simulink model "ES105A_StHlthSigNormn"  (R2013b)
settings: Solver=FixedStepDiscrete  SolverMode=SingleTasking  StartTime=0.0  StopTime=1  FixedStep=0.002  RelTol=1e-3
undefined symbols (not defined in the file): ARCHGLBPRM_FLOATZEROTHD_ULS_F32, CurrMeasCorrlnMaxErrCurr, CURRMOTSUMDIVBYZEROPROTNVAL_AMPR_F32, DIGTQDIVBYZEROPROTNVAL_HWNWTMTR_F32, DutyCycThermProtnDutyCycFildThd, EcuTMeasRngDiagcMax, EcuTMeasRngDiagcMin, EotLrngAuthyStrtLrn, FRICESTIMNDIVBYZEROPROTNVAL_HWNWTMTR_F32, HLTH0PERC_CNT_U08, HLTH100PERC_CNT_F32, HLTH100PERC_CNT_U08, HLTH50PERC_CNT_U08, HwTqCorrlnChATraSumSetFltThd, HwTqCorrlnChBTraSumSetFltThd, HWTQIDPTSIG_CNT_U08, MOTAG2MEAS_VALMAXERR_VOLTSQD_F32, MOTAG2MEAS_VALMINERR_VOLTSQD_F32, MOTAGCORRLN_MOTAGCORRLNERRTHD_MOTREVELEC_U0P16, MotDrvDiagcErrThd, MOTPOS2DIVBYZEROPROTNVAL2_VOLTSQD_F32, MOTPOS2DIVBYZEROPROTNVAL_VOLTSQD_F32, MOTPOSNERRDIVBYZEROPROTNVAL_MOTREV_U16, MOTPOSNERRZEROTHD_MOTREV_U0P16, NtcNr1, NtcSts1, PHAVLTGDIVBYZEROPROTNVAL_NANOSEC_F32, SigQlfr1, STHLTHSCAGFAC_CNT_F32, StHlthSigNormnAbsltMotPosDifStHlthDiagThd, StHlthSigNormnCurrMotSumStHlthDiagThd, StHlthSigNormnDigTqStHlthDiagThd, StHlthSigNormnDutyCycFltLimThd, StHlthSigNormnHiCtrlrT, StHlthSigNormnIdptSigStHlthSca, StHlthSigNormnLoCtrlrT, StHlthSigNormnMaxFricThd, StHlthSigNormnMinRackTrvlLim, StHlthSigNormnMotPosStHlthDiagThd, StHlthSigNormnMotVelCal, StHlthSigNormnPhaInfoStHlthDiagThd, StHlthSigNormnStHlthCorrlnErr, StHlthSigNormnStHlthCurrMotSum, StHlthSigNormnStHlthPhaInfo, StHlthSigNormnValMaxStHlthErr, StHlthSigNormnValMinStHlthErr, StHlthSigNormnWhlImbRejctnThd, SysGlbPrmMotPoleCnt, TSTHLTH0PERC_CNT_U08, u2, u3, u4, VLTGSTHLTH0PERC_CNT_U08
libraries: NxtrLim x39, simulink x33, NxtrAbslt x4
(part 3 of 10)

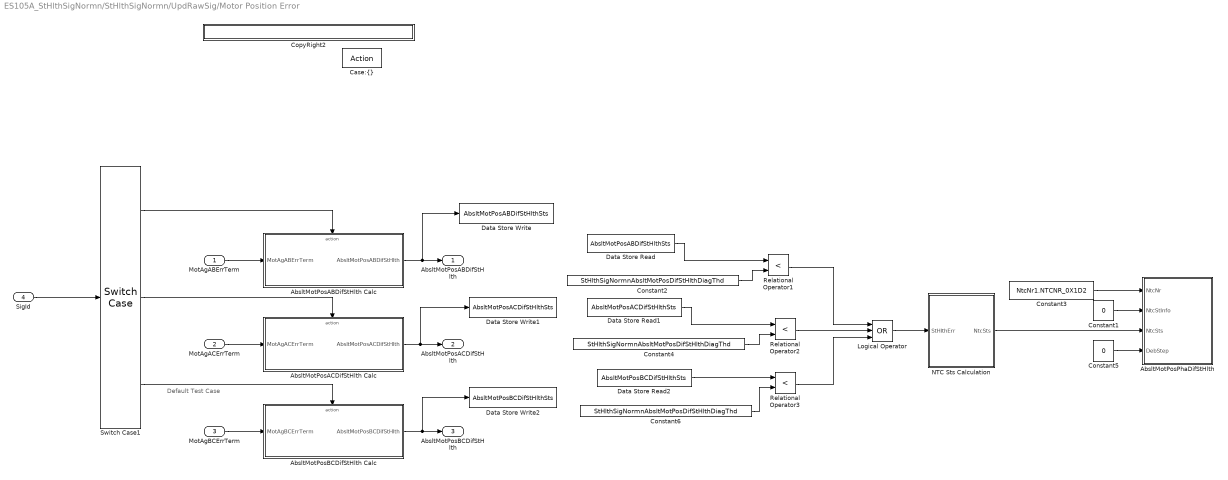
== system ES105A_StHlthSigNormn/StHlthSigNormn/UpdRawSig/Motor Position Error  ==
  note: Default Test Case
  MotAgABErrTerm : Inport
  MotAgACErrTerm : Inport  Port=2
  MotAgBCErrTerm : Inport  Port=3
  SigId : Inport  Port=4
  "Case:{}" : ActionPort  ActionType=case
  AbsltMotPosABDifStHlth Calc : Subsystem  TreatAsAtomicUnit=on
  AbsltMotPosACDifStHlth Calc : Subsystem  TreatAsAtomicUnit=on
  AbsltMotPosBCDifStHlth Calc : Subsystem  TreatAsAtomicUnit=on
  AbsltMotPosPhaDifStHlth : Subsystem  mask(SetNTC){}
      mask help: SetNTC library block
  Constant1 : Constant  Value=0  OutDataTypeStr=uint8
      settings: AttributesFormatString=%<OutDataTypeStr>
  Constant2 : Constant  Value=StHlthSigNormnAbsltMotPosDifStHlthDiagThd
  Constant3 : Constant  Value=NtcNr1.NTCNR_0X1D2  OutDataTypeStr=Enum: NtcNr1
  Constant4 : Constant  Value=StHlthSigNormnAbsltMotPosDifStHlthDiagThd
  Constant5 : Constant  Value=0  OutDataTypeStr=uint16
      settings: AttributesFormatString=%<OutDataTypeStr>
  Constant6 : Constant  Value=StHlthSigNormnAbsltMotPosDifStHlthDiagThd
  CopyRight2 : Subsystem  Description=|  mask(Copyright Information){none=on}
      | Copyright info block.                                               
      |                                                                     
      | Place copyright information at the top of every subsystem in design.
      mask prompts: none "No parameters"
      mask help: Place copyright information at the top of every subsystem in design.
      mask Display:
      | NxtrConf = 'Nexteer Confidential';
      | 
      | sys = bdroot; %handle for the current model ("system")
      | first = get_param(sys,'Created');
      | first = first(end-3:end);  %year is last four digits
      | 
      | last = get_param(sys,'LastModifiedDate');
      | if isempty(last)
      |     last = datestr(now,'yyyy');
      | else
      |     last = last(end-3:end);
      | end
      | 
      | if strcmp(first,last)
      |     fprintf('%s -- Copyright %s Nexteer',NxtrConf,first)
      | else
      |     fprintf('%s -- %s%s- %s Nexteer',NxtrConf,char(169),first,last)
      | end
  Data Store Read : DataStoreRead  DataStoreName=AbsltMotPosABDifStHlthSts
  Data Store Read1 : DataStoreRead  DataStoreName=AbsltMotPosACDifStHlthSts
  Data Store Read2 : DataStoreRead  DataStoreName=AbsltMotPosBCDifStHlthSts
  Data Store Write : DataStoreWrite  DataStoreName=AbsltMotPosABDifStHlthSts
  Data Store Write1 : DataStoreWrite  DataStoreName=AbsltMotPosACDifStHlthSts
  Data Store Write2 : DataStoreWrite  DataStoreName=AbsltMotPosBCDifStHlthSts
  Logical Operator : Logic  Operator=OR  Inputs=3  AllPortsSameDT=off  OutDataTypeStr=boolean
  NTC Sts Calculation : Subsystem
  Relational Operator1 : RelationalOperator  Operator=<  OutDataTypeStr=boolean
  Relational Operator2 : RelationalOperator  Operator=<  OutDataTypeStr=boolean
  Relational Operator3 : RelationalOperator  Operator=<  OutDataTypeStr=boolean
  Switch Case1 : SwitchCase  CaseConditions={StHlthMonSig3.STHLTHMONSIG_MOTPOSABDIFF, StHlthMonSig3.STHLTHMONSIG_MOTPOSACDIFF}
  AbsltMotPosABDifStHlth : Outport
  AbsltMotPosACDifStHlth : Outport  Port=2
  AbsltMotPosBCDifStHlth : Outport  Port=3
  wires:
  Constant3/1 -> AbsltMotPosPhaDifStHlth/1(NtcNr)
  Constant1/1 -> AbsltMotPosPhaDifStHlth/2(NtcStInfo)
  Constant5/1 -> AbsltMotPosPhaDifStHlth/4(DebStep)
  NTC Sts Calculation/1(NtcSts) -> AbsltMotPosPhaDifStHlth/3(NtcSts)
  AbsltMotPosACDifStHlth Calc/1(AbsltMotPosACDifStHlth) -> Data Store Write1/1, AbsltMotPosACDifStHlth/1
  Switch Case1/1 -> AbsltMotPosABDifStHlth Calc/Action
  MotAgABErrTerm/1 -> AbsltMotPosABDifStHlth Calc/1(MotAgABErrTerm)
  Switch Case1/2 -> AbsltMotPosACDifStHlth Calc/Action
  MotAgACErrTerm/1 -> AbsltMotPosACDifStHlth Calc/1(MotAgACErrTerm)
  Switch Case1/3 -> AbsltMotPosBCDifStHlth Calc/Action
  MotAgBCErrTerm/1 -> AbsltMotPosBCDifStHlth Calc/1(MotAgBCErrTerm)
  SigId/1 -> Switch Case1/1
  AbsltMotPosABDifStHlth Calc/1(AbsltMotPosABDifStHlth) -> Data Store Write/1, AbsltMotPosABDifStHlth/1
  AbsltMotPosBCDifStHlth Calc/1(AbsltMotPosBCDifStHlth) -> Data Store Write2/1, AbsltMotPosBCDifStHlth/1
  Constant2/1 -> Relational Operator1/2
  Data Store Read/1 -> Relational Operator1/1
  Constant4/1 -> Relational Operator2/2
  Data Store Read1/1 -> Relational Operator2/1
  Constant6/1 -> Relational Operator3/2
  Data Store Read2/1 -> Relational Operator3/1
  Relational Operator1/1 -> Logical Operator/1
  Relational Operator2/1 -> Logical Operator/2
  Relational Operator3/1 -> Logical Operator/3
  Logical Operator/1 -> NTC Sts Calculation/1(StHlthErr)

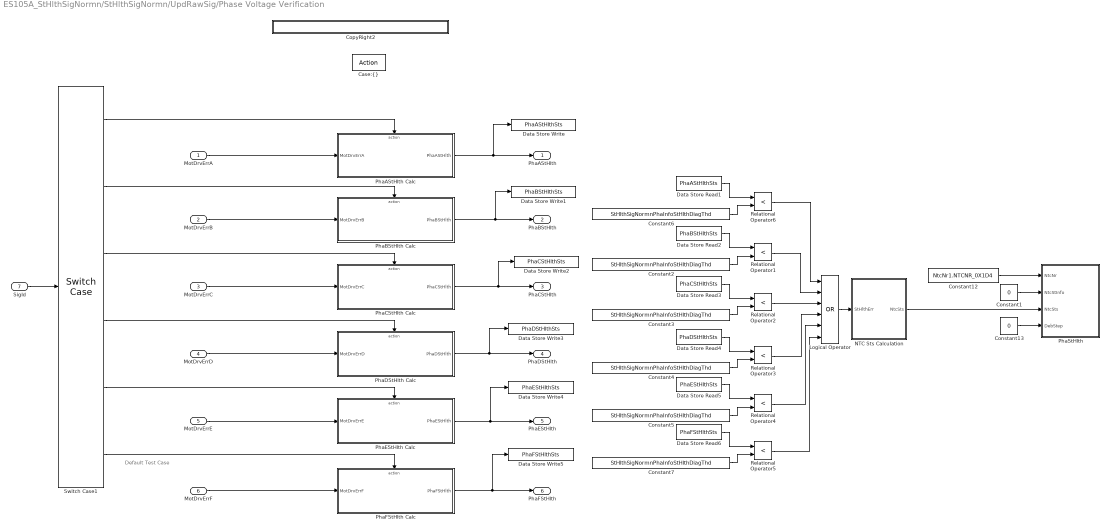
== system ES105A_StHlthSigNormn/StHlthSigNormn/UpdRawSig/Phase Voltage Verification ==
  note: Default Test Case
  MotDrvErrA : Inport
  MotDrvErrB : Inport  Port=2
  MotDrvErrC : Inport  Port=3
  MotDrvErrD : Inport  Port=4
  MotDrvErrE : Inport  Port=5
  MotDrvErrF : Inport  Port=6
  SigId : Inport  Port=7
  "Case:{}" : ActionPort  ActionType=case
  Constant1 : Constant  Value=0  OutDataTypeStr=uint8
      settings: AttributesFormatString=%<OutDataTypeStr>
  Constant12 : Constant  Value=NtcNr1.NTCNR_0X1D4  OutDataTypeStr=Enum: NtcNr1
  Constant13 : Constant  Value=0  OutDataTypeStr=uint16
      settings: AttributesFormatString=%<OutDataTypeStr>
  Constant{2..7} (6 alike) : Constant  Value=StHlthSigNormnPhaInfoStHlthDiagThd
  CopyRight2 : Subsystem  Description=|  mask(Copyright Information){none=on}
      | Copyright info block.                                               
      |                                                                     
      | Place copyright information at the top of every subsystem in design.
      mask prompts: none "No parameters"
      mask help: Place copyright information at the top of every subsystem in design.
      mask Display:
      | NxtrConf = 'Nexteer Confidential';
      | 
      | sys = bdroot; %handle for the current model ("system")
      | first = get_param(sys,'Created');
      | first = first(end-3:end);  %year is last four digits
      | 
      | last = get_param(sys,'LastModifiedDate');
      | if isempty(last)
      |     last = datestr(now,'yyyy');
      | else
      |     last = last(end-3:end);
      | end
      | 
      | if strcmp(first,last)
      |     fprintf('%s -- Copyright %s Nexteer',NxtrConf,first)
      | else
      |     fprintf('%s -- %s%s- %s Nexteer',NxtrConf,char(169),first,last)
      | end
  Data Store Read1 : DataStoreRead  DataStoreName=PhaAStHlthSts
  Data Store Read2 : DataStoreRead  DataStoreName=PhaBStHlthSts
  Data Store Read3 : DataStoreRead  DataStoreName=PhaCStHlthSts
  Data Store Read4 : DataStoreRead  DataStoreName=PhaDStHlthSts
  Data Store Read5 : DataStoreRead  DataStoreName=PhaEStHlthSts
  Data Store Read6 : DataStoreRead  DataStoreName=PhaFStHlthSts
  Data Store Write : DataStoreWrite  DataStoreName=PhaAStHlthSts
  Data Store Write1 : DataStoreWrite  DataStoreName=PhaBStHlthSts
  Data Store Write2 : DataStoreWrite  DataStoreName=PhaCStHlthSts
  Data Store Write3 : DataStoreWrite  DataStoreName=PhaDStHlthSts
  Data Store Write4 : DataStoreWrite  DataStoreName=PhaEStHlthSts
  Data Store Write5 : DataStoreWrite  DataStoreName=PhaFStHlthSts
  Logical Operator : Logic  Operator=OR  Inputs=6  AllPortsSameDT=off  OutDataTypeStr=boolean
  NTC Sts Calculation : Subsystem
  PhaAStHlth Calc : Subsystem  TreatAsAtomicUnit=on
  PhaBStHlth Calc : Subsystem  TreatAsAtomicUnit=on
  PhaCStHlth Calc : Subsystem  TreatAsAtomicUnit=on
  PhaDStHlth Calc : Subsystem  TreatAsAtomicUnit=on
  PhaEStHlth Calc : Subsystem  TreatAsAtomicUnit=on
  PhaFStHlth Calc : Subsystem  TreatAsAtomicUnit=on
  PhaStHlth : Subsystem  mask(SetNTC){}
      mask help: SetNTC library block
  Relational Operator{1..6} (6 alike) : RelationalOperator  Operator=<  OutDataTypeStr=boolean
  Switch Case1 : SwitchCase  CaseConditions={StHlthMonSig3.STHLTHMONSIG_MOTPOSPHASEA,StHlthMonSig3.STHLTHMONSIG_MOTPOSPHASEB,StHlthMonSig3.STHLTHMONSIG_MOTPOSPHASEC,StHlthMonSig3.STHLTHMONSIG_MOTPOSPHASED,StHlthMonSig3.STHLTHMONSIG_MOTPOSPHASEE}
  PhaAStHlth : Outport
  PhaBStHlth : Outport  Port=2
  PhaCStHlth : Outport  Port=3
  PhaDStHlth : Outport  Port=4
  PhaEStHlth : Outport  Port=5
  PhaFStHlth : Outport  Port=6
  wires:
  Constant12/1 -> PhaStHlth/1(NtcNr)
  Constant1/1 -> PhaStHlth/2(NtcStInfo)
  Constant13/1 -> PhaStHlth/4(DebStep)
  NTC Sts Calculation/1(NtcSts) -> PhaStHlth/3(NtcSts)
  MotDrvErrA/1 -> PhaAStHlth Calc/1(MotDrvErrA)
  MotDrvErrB/1 -> PhaBStHlth Calc/1(MotDrvErrB)
  MotDrvErrC/1 -> PhaCStHlth Calc/1(MotDrvErrC)
  MotDrvErrD/1 -> PhaDStHlth Calc/1(MotDrvErrD)
  MotDrvErrE/1 -> PhaEStHlth Calc/1(MotDrvErrE)
  MotDrvErrF/1 -> PhaFStHlth Calc/1(MotDrvErrF)
  Switch Case1/1 -> PhaAStHlth Calc/Action
  Switch Case1/2 -> PhaBStHlth Calc/Action
  Switch Case1/3 -> PhaCStHlth Calc/Action
  Switch Case1/4 -> PhaDStHlth Calc/Action
  Switch Case1/5 -> PhaEStHlth Calc/Action
  Switch Case1/6 -> PhaFStHlth Calc/Action
  SigId/1 -> Switch Case1/1
  PhaEStHlth Calc/1(PhaEStHlth) -> Data Store Write4/1, PhaEStHlth/1
  PhaAStHlth Calc/1(PhaAStHlth) -> Data Store Write/1, PhaAStHlth/1
  PhaBStHlth Calc/1(PhaBStHlth) -> Data Store Write1/1, PhaBStHlth/1
  PhaCStHlth Calc/1(PhaCStHlth) -> Data Store Write2/1, PhaCStHlth/1
  PhaDStHlth Calc/1(PhaDStHlth) -> Data Store Write3/1, PhaDStHlth/1
  PhaFStHlth Calc/1(PhaFStHlth) -> Data Store Write5/1, PhaFStHlth/1
  Constant6/1 -> Relational Operator6/2
  Data Store Read1/1 -> Relational Operator6/1
  Constant2/1 -> Relational Operator1/2
  Data Store Read2/1 -> Relational Operator1/1
  Constant3/1 -> Relational Operator2/2
  Data Store Read3/1 -> Relational Operator2/1
  Constant4/1 -> Relational Operator3/2
  Data Store Read4/1 -> Relational Operator3/1
  Constant5/1 -> Relational Operator4/2
  Data Store Read5/1 -> Relational Operator4/1
  Constant7/1 -> Relational Operator5/2
  Data Store Read6/1 -> Relational Operator5/1
  Relational Operator1/1 -> Logical Operator/2
  Relational Operator6/1 -> Logical Operator/1
  Relational Operator2/1 -> Logical Operator/3
  Relational Operator3/1 -> Logical Operator/4
  Relational Operator4/1 -> Logical Operator/5
  Relational Operator5/1 -> Logical Operator/6
  Logical Operator/1 -> NTC Sts Calculation/1(StHlthErr)

== system ES105A_StHlthSigNormn/StHlthSigNormn/UpdRawSig/Single Bit Correction  ==
  note: Datatype conversion is added to avoid simulation error as
      | Uint8 is expected at the input of saturation block
  LclRamEccSngBitCntrOutp : Inport
  "Case:{}" : ActionPort  ActionType=case
  Constant : Constant  Value=STHLTHSCAGFAC_CNT_F32  OutDataTypeStr=single
  CopyRight2 : Subsystem  Description=|  mask(Copyright Information){none=on}
      | Copyright info block.                                               
      |                                                                     
      | Place copyright information at the top of every subsystem in design.
      mask prompts: none "No parameters"
      mask help: Place copyright information at the top of every subsystem in design.
      mask Display:
      | NxtrConf = 'Nexteer Confidential';
      | 
      | sys = bdroot; %handle for the current model ("system")
      | first = get_param(sys,'Created');
      | first = first(end-3:end);  %year is last four digits
      | 
      | last = get_param(sys,'LastModifiedDate');
      | if isempty(last)
      |     last = datestr(now,'yyyy');
      | else
      |     last = last(end-3:end);
      | end
      | 
      | if strcmp(first,last)
      |     fprintf('%s -- Copyright %s Nexteer',NxtrConf,first)
      | else
      |     fprintf('%s -- %s%s- %s Nexteer',NxtrConf,char(169),first,last)
      | end
  Data Type Conversion : DataTypeConversion  OutDataTypeStr=uint8
  LimStat_u2 : NxtrLim/LimStat_u08  LoLim=RamEccSngBitCorrnStHlth.EngMin  HiLim=RamEccSngBitCorrnStHlth.EngMax
      settings: AttributesFormatString=|
      | Low Limit: %<LoLim>
      | High Limit:%<HiLim>
  Subtract : Sum  Inputs=+-
  RamEccSngBitCorrnStHlth : Outport
  wires:
  Constant/1 -> Data Type Conversion/1
  LclRamEccSngBitCntrOutp/1 -> Subtract/2
  Subtract/1 -> LimStat_u2/1
  LimStat_u2/1 -> RamEccSngBitCorrnStHlth/1
  Data Type Conversion/1 -> Subtract/1

== system ES105A_StHlthSigNormn/StHlthSigNormn/UpdRawSig/Wheel Imbalance Rejection ==
  WhlImbRejctnCmd : Inport
  "Case:{}" : ActionPort  ActionType=case
  Abs : Abs
  Constant : Constant  Value=StHlthSigNormnWhlImbRejctnThd
  CopyRight2 : Subsystem  Description=|  mask(Copyright Information){none=on}
      | Copyright info block.                                               
      |                                                                     
      | Place copyright information at the top of every subsystem in design.
      mask prompts: none "No parameters"
      mask help: Place copyright information at the top of every subsystem in design.
      mask Display:
      | NxtrConf = 'Nexteer Confidential';
      | 
      | sys = bdroot; %handle for the current model ("system")
      | first = get_param(sys,'Created');
      | first = first(end-3:end);  %year is last four digits
      | 
      | last = get_param(sys,'LastModifiedDate');
      | if isempty(last)
      |     last = datestr(now,'yyyy');
      | else
      |     last = last(end-3:end);
      | end
      | 
      | if strcmp(first,last)
      |     fprintf('%s -- Copyright %s Nexteer',NxtrConf,first)
      | else
      |     fprintf('%s -- %s%s- %s Nexteer',NxtrConf,char(169),first,last)
      | end
  If : If  IfExpression=u1
  If Action Subsystem : Subsystem  TreatAsAtomicUnit=on
  If Action Subsystem2 : Subsystem  TreatAsAtomicUnit=on
  LimStat_u2 : NxtrLim/LimStat_u08  LoLim=WHLIMBMAXCMPSTHLTHLOLI_CNT_U08  HiLim=WHLIMBMAXCMPSTHLTHHILI_CNT_U08
      settings: AttributesFormatString=|
      | Low Limit: %<LoLim>
      | High Limit:%<HiLim>
  Merge : Merge
  Relational Operator : RelationalOperator  OutDataTypeStr=boolean
  WhlImbMaxCmpStHlth : Outport
  wires:
  Constant/1 -> Relational Operator/2
  Relational Operator/1 -> If/1
  If/1 -> If Action Subsystem/Action
  WhlImbRejctnCmd/1 -> Abs/1
  If/2 -> If Action Subsystem2/Action
  If Action Subsystem/1(WhlImbMaxCmpStHlth) -> Merge/1
  If Action Subsystem2/1(WhlImbMaxCmpStHlth) -> Merge/2
  Merge/1 -> LimStat_u2/1
  LimStat_u2/1 -> WhlImbMaxCmpStHlth/1
  Abs/1 -> Relational Operator/1

== system ES105A_StHlthSigNormn/StHlthSigNormn/StHlthSigNormnInit1/GetFricLrngData/CopyRight2 ==

== system ES105A_StHlthSigNormn/StHlthSigNormn/StHlthSigNormnInit1/Motror Angle Threshold Calc/CopyRight2 ==

== system ES105A_StHlthSigNormn/StHlthSigNormn/UpdRawSig/ EOT Impact Counter/CopyRight2 ==

== system ES105A_StHlthSigNormn/StHlthSigNormn/UpdRawSig/ EOT Impact Counter/If Action Subsystem ==
  HwAg : Inport
  RackLimrEotSig0Avl : Inport  Port=2
  MotVelCrf : Inport  Port=3
  HwAgEotCcw : Inport  Port=4
  RackLimrEotSig1Avl : Inport  Port=5
  HwAgEotCw : Inport  Port=6
  Action Port : ActionPort  ActionType=then
  Constant : Constant  Value=ARCHGLBPRM_FLOATZEROTHD_ULS_F32
  CopyRight2 : Subsystem  Description=|  mask(Copyright Information){none=on}
      | Copyright info block.                                               
      |                                                                     
      | Place copyright information at the top of every subsystem in design.
      mask prompts: none "No parameters"
      mask help: Place copyright information at the top of every subsystem in design.
      mask Display:
      | NxtrConf = 'Nexteer Confidential';
      | 
      | sys = bdroot; %handle for the current model ("system")
      | first = get_param(sys,'Created');
      | first = first(end-3:end);  %year is last four digits
      | 
      | last = get_param(sys,'LastModifiedDate');
      | if isempty(last)
      |     last = datestr(now,'yyyy');
      | else
      |     last = last(end-3:end);
      | end
      | 
      | if strcmp(first,last)
      |     fprintf('%s -- Copyright %s Nexteer',NxtrConf,first)
      | else
      |     fprintf('%s -- %s%s- %s Nexteer',NxtrConf,char(169),first,last)
      | end
  If : If  IfExpression=u1
  If Action Subsystem : Subsystem  TreatAsAtomicUnit=on
  If Action Subsystem1 : Subsystem  TreatAsAtomicUnit=on
  Relational Operator : RelationalOperator  OutDataTypeStr=boolean
  wires:
  HwAg/1 -> Relational Operator/1, [HwAg]
  Constant/1 -> Relational Operator/2
  Relational Operator/1 -> If/1
  If/1 -> If Action Subsystem/Action
  RackLimrEotSig1Avl/1 -> If Action Subsystem/1(RackLimrEotSig1Avl)
  HwAgEotCw/1 -> If Action Subsystem/4(HwAgEotCw)
  If/2 -> If Action Subsystem1/Action
  MotVelCrf/1 -> [MotVelCrf], If Action Subsystem1/3(MotVelCrf)
  RackLimrEotSig0Avl/1 -> If Action Subsystem1/1(RackLimrEotSig0Avl)
  HwAgEotCcw/1 -> If Action Subsystem1/4(HwAgEotCcw)
  [MotVelCrf] -> If Action Subsystem/3("MotVelCrf ")
  [HwAg] -> If Action Subsystem/2(HwAg)
  [HwAg] -> If Action Subsystem1/2(HwAg)

== system ES105A_StHlthSigNormn/StHlthSigNormn/UpdRawSig/ EOT Impact Counter/If Action Subsystem1 ==
  Action Port : ActionPort  ActionType=else
  Constant : Constant  Value=0  OutDataTypeStr=boolean
      settings: AttributesFormatString=%<OutDataTypeStr>
  CopyRight2 : Subsystem  Description=|  mask(Copyright Information){none=on}
      | Copyright info block.                                               
      |                                                                     
      | Place copyright information at the top of every subsystem in design.
      mask prompts: none "No parameters"
      mask help: Place copyright information at the top of every subsystem in design.
      mask Display:
      | NxtrConf = 'Nexteer Confidential';
      | 
      | sys = bdroot; %handle for the current model ("system")
      | first = get_param(sys,'Created');
      | first = first(end-3:end);  %year is last four digits
      | 
      | last = get_param(sys,'LastModifiedDate');
      | if isempty(last)
      |     last = datestr(now,'yyyy');
      | else
      |     last = last(end-3:end);
      | end
      | 
      | if strcmp(first,last)
      |     fprintf('%s -- Copyright %s Nexteer',NxtrConf,first)
      | else
      |     fprintf('%s -- %s%s- %s Nexteer',NxtrConf,char(169),first,last)
      | end
  Data Store Write : DataStoreWrite  DataStoreName=EntrEot
  wires:
  Constant/1 -> Data Store Write/1

== system ES105A_StHlthSigNormn/StHlthSigNormn/UpdRawSig/ Health Of Assist Due To Voltage/CopyRight2 ==

== system ES105A_StHlthSigNormn/StHlthSigNormn/UpdRawSig/ Health Of Assist Due To Voltage/Do nothing ==
  Action Port : ActionPort  ActionType=else
  CopyRight2 : Subsystem  Description=|  mask(Copyright Information){none=on}
      | Copyright info block.                                               
      |                                                                     
      | Place copyright information at the top of every subsystem in design.
      mask prompts: none "No parameters"
      mask help: Place copyright information at the top of every subsystem in design.
      mask Display:
      | NxtrConf = 'Nexteer Confidential';
      | 
      | sys = bdroot; %handle for the current model ("system")
      | first = get_param(sys,'Created');
      | first = first(end-3:end);  %year is last four digits
      | 
      | last = get_param(sys,'LastModifiedDate');
      | if isempty(last)
      |     last = datestr(now,'yyyy');
      | else
      |     last = last(end-3:end);
      | end
      | 
      | if strcmp(first,last)
      |     fprintf('%s -- Copyright %s Nexteer',NxtrConf,first)
      | else
      |     fprintf('%s -- %s%s- %s Nexteer',NxtrConf,char(169),first,last)
      | end

== system ES105A_StHlthSigNormn/StHlthSigNormn/UpdRawSig/ Health Of Assist Due To Voltage/LowVoltage ==
  Action Port : ActionPort  ActionType=elseif
  Bitwise Operator : simulink/Logic and Bit Operations/Bitwise Operator  logicop=OR  UseBitMask=off  NumInputPorts=2  BitMask=bin2dec('11011001')  BitMaskRealWorld=Stored Integer
  Constant1 : Constant  Value=HLTH50PERC_CNT_U08  OutDataTypeStr=uint8
  Constant2 : Constant  OutDataTypeStr=uint8
      settings: AttributesFormatString=%<OutDataTypeStr>
  Constant3 : Constant  OutDataTypeStr=uint8
      settings: AttributesFormatString=%<OutDataTypeStr>
  CopyRight2 : Subsystem  Description=|  mask(Copyright Information){none=on}
      | Copyright info block.                                               
      |                                                                     
      | Place copyright information at the top of every subsystem in design.
      mask prompts: none "No parameters"
      mask help: Place copyright information at the top of every subsystem in design.
      mask Display:
      | NxtrConf = 'Nexteer Confidential';
      | 
      | sys = bdroot; %handle for the current model ("system")
      | first = get_param(sys,'Created');
      | first = first(end-3:end);  %year is last four digits
      | 
      | last = get_param(sys,'LastModifiedDate');
      | if isempty(last)
      |     last = datestr(now,'yyyy');
      | else
      |     last = last(end-3:end);
      | end
      | 
      | if strcmp(first,last)
      |     fprintf('%s -- Copyright %s Nexteer',NxtrConf,first)
      | else
      |     fprintf('%s -- %s%s- %s Nexteer',NxtrConf,char(169),first,last)
      | end
  Data Store Read : DataStoreRead  DataStoreName=VltgRngIgnCyc
  Data Store Write : DataStoreWrite  DataStoreName=VltgRngIgnCyc
  Shift Arithmetic : ArithShift  BitShiftNumber=LOVLTGSTHLTH50PERC_CNT_U08  BitShiftDirection=Left
  Shift Arithmetic1 : ArithShift  BitShiftNumber=LOVLTGSTHLTH50PERC_CNT_U08  BitShiftDirection=Left
  OutpAssiStHlth : Outport
  " PrsntVltgRng" : Outport  Port=2
  wires:
  Constant1/1 -> OutpAssiStHlth/1
  Constant2/1 -> Shift Arithmetic/1
  Shift Arithmetic/1 -> Bitwise Operator/2
  Data Store Read/1 -> Bitwise Operator/1
  Bitwise Operator/1 -> Data Store Write/1
  Constant3/1 -> Shift Arithmetic1/1
  Shift Arithmetic1/1 -> " PrsntVltgRng"/1

== system ES105A_StHlthSigNormn/StHlthSigNormn/UpdRawSig/ Health Of Assist Due To Voltage/NtcLoVltgActvSts ==
  NtcNr : Inport
  CopyRight2 : Subsystem  Description=|  mask(Copyright Information){none=on}
      | Copyright info block.                                               
      |                                                                     
      | Place copyright information at the top of every subsystem in design.
      mask prompts: none "No parameters"
      mask help: Place copyright information at the top of every subsystem in design.
      mask Display:
      | NxtrConf = 'Nexteer Confidential';
      | 
      | sys = bdroot; %handle for the current model ("system")
      | first = get_param(sys,'Created');
      | first = first(end-3:end);  %year is last four digits
      | 
      | last = get_param(sys,'LastModifiedDate');
      | if isempty(last)
      |     last = datestr(now,'yyyy');
      | else
      |     last = last(end-3:end);
      | end
      | 
      | if strcmp(first,last)
      |     fprintf('%s -- Copyright %s Nexteer',NxtrConf,first)
      | else
      |     fprintf('%s -- %s%s- %s Nexteer',NxtrConf,char(169),first,last)
      | end
  Data Store Read : DataStoreRead  DataStoreName=Ntc0X0B1Qlfr
  Terminator : Terminator
  Ntc0X0B1Qlfr : Outport
  wires:
  NtcNr/1 -> Terminator/1
  Data Store Read/1 -> Ntc0X0B1Qlfr/1

== system ES105A_StHlthSigNormn/StHlthSigNormn/UpdRawSig/ Health Of Assist Due To Voltage/NtcOverVltgActvSts ==
  NtcNr : Inport
  CopyRight2 : Subsystem  Description=|  mask(Copyright Information){none=on}
      | Copyright info block.                                               
      |                                                                     
      | Place copyright information at the top of every subsystem in design.
      mask prompts: none "No parameters"
      mask help: Place copyright information at the top of every subsystem in design.
      mask Display:
      | NxtrConf = 'Nexteer Confidential';
      | 
      | sys = bdroot; %handle for the current model ("system")
      | first = get_param(sys,'Created');
      | first = first(end-3:end);  %year is last four digits
      | 
      | last = get_param(sys,'LastModifiedDate');
      | if isempty(last)
      |     last = datestr(now,'yyyy');
      | else
      |     last = last(end-3:end);
      | end
      | 
      | if strcmp(first,last)
      |     fprintf('%s -- Copyright %s Nexteer',NxtrConf,first)
      | else
      |     fprintf('%s -- %s%s- %s Nexteer',NxtrConf,char(169),first,last)
      | end
  Data Store Read : DataStoreRead  DataStoreName=Ntc0X0B5Qlfr
  Terminator : Terminator
  Ntc0X0B5Qlfr : Outport
  wires:
  Data Store Read/1 -> Ntc0X0B5Qlfr/1
  NtcNr/1 -> Terminator/1

== system ES105A_StHlthSigNormn/StHlthSigNormn/UpdRawSig/ Health Of Assist Due To Voltage/NtcUnderVltgActvSts ==
  NtcNr : Inport
  CopyRight2 : Subsystem  Description=|  mask(Copyright Information){none=on}
      | Copyright info block.                                               
      |                                                                     
      | Place copyright information at the top of every subsystem in design.
      mask prompts: none "No parameters"
      mask help: Place copyright information at the top of every subsystem in design.
      mask Display:
      | NxtrConf = 'Nexteer Confidential';
      | 
      | sys = bdroot; %handle for the current model ("system")
      | first = get_param(sys,'Created');
      | first = first(end-3:end);  %year is last four digits
      | 
      | last = get_param(sys,'LastModifiedDate');
      | if isempty(last)
      |     last = datestr(now,'yyyy');
      | else
      |     last = last(end-3:end);
      | end
      | 
      | if strcmp(first,last)
      |     fprintf('%s -- Copyright %s Nexteer',NxtrConf,first)
      | else
      |     fprintf('%s -- %s%s- %s Nexteer',NxtrConf,char(169),first,last)
      | end
  Data Store Read : DataStoreRead  DataStoreName=Ntc0X0B0Qlfr
  Terminator : Terminator
  Ntc0X0B0Qlfr : Outport
  wires:
  NtcNr/1 -> Terminator/1
  Data Store Read/1 -> Ntc0X0B0Qlfr/1

== system ES105A_StHlthSigNormn/StHlthSigNormn/UpdRawSig/ Health Of Assist Due To Voltage/OverVoltage ==
  Action Port : ActionPort  ActionType=elseif
  Bitwise Operator : simulink/Logic and Bit Operations/Bitwise Operator  logicop=OR  UseBitMask=off  NumInputPorts=2  BitMask=bin2dec('11011001')  BitMaskRealWorld=Stored Integer
  Constant1 : Constant  Value=HLTH0PERC_CNT_U08  OutDataTypeStr=uint8
      settings: AttributesFormatString=%<OutDataTypeStr>
  Constant2 : Constant  OutDataTypeStr=uint8
      settings: AttributesFormatString=%<OutDataTypeStr>
  Constant3 : Constant  OutDataTypeStr=uint8
      settings: AttributesFormatString=%<OutDataTypeStr>
  CopyRight2 : Subsystem  Description=|  mask(Copyright Information){none=on}
      | Copyright info block.                                               
      |                                                                     
      | Place copyright information at the top of every subsystem in design.
      mask prompts: none "No parameters"
      mask help: Place copyright information at the top of every subsystem in design.
      mask Display:
      | NxtrConf = 'Nexteer Confidential';
      | 
      | sys = bdroot; %handle for the current model ("system")
      | first = get_param(sys,'Created');
      | first = first(end-3:end);  %year is last four digits
      | 
      | last = get_param(sys,'LastModifiedDate');
      | if isempty(last)
      |     last = datestr(now,'yyyy');
      | else
      |     last = last(end-3:end);
      | end
      | 
      | if strcmp(first,last)
      |     fprintf('%s -- Copyright %s Nexteer',NxtrConf,first)
      | else
      |     fprintf('%s -- %s%s- %s Nexteer',NxtrConf,char(169),first,last)
      | end
  Data Store Read : DataStoreRead  DataStoreName=VltgRngIgnCyc
  Data Store Write : DataStoreWrite  DataStoreName=VltgRngIgnCyc
  Shift Arithmetic : ArithShift  BitShiftNumber=HIVLTGSTHLTH0PERC_CNT_U08  BitShiftDirection=Left
  Shift Arithmetic1 : ArithShift  BitShiftNumber=HIVLTGSTHLTH0PERC_CNT_U08  BitShiftDirection=Left
  OutpAssiStHlth : Outport
  " PrsntVltgRng" : Outport  Port=2
  wires:
  Constant1/1 -> OutpAssiStHlth/1
  Constant2/1 -> Shift Arithmetic/1
  Shift Arithmetic/1 -> Bitwise Operator/2
  Data Store Read/1 -> Bitwise Operator/1
  Bitwise Operator/1 -> Data Store Write/1
  Constant3/1 -> Shift Arithmetic1/1
  Shift Arithmetic1/1 -> " PrsntVltgRng"/1

== system ES105A_StHlthSigNormn/StHlthSigNormn/UpdRawSig/ Health Of Assist Due To Voltage/Safe Operating Conditions ==
  Action Port : ActionPort  ActionType=then
  Constant1 : Constant  Value=HLTH100PERC_CNT_U08  OutDataTypeStr=uint8
  Constant3 : Constant  Value=0  OutDataTypeStr=uint8
      settings: AttributesFormatString=%<OutDataTypeStr>
  CopyRight2 : Subsystem  Description=|  mask(Copyright Information){none=on}
      | Copyright info block.                                               
      |                                                                     
      | Place copyright information at the top of every subsystem in design.
      mask prompts: none "No parameters"
      mask help: Place copyright information at the top of every subsystem in design.
      mask Display:
      | NxtrConf = 'Nexteer Confidential';
      | 
      | sys = bdroot; %handle for the current model ("system")
      | first = get_param(sys,'Created');
      | first = first(end-3:end);  %year is last four digits
      | 
      | last = get_param(sys,'LastModifiedDate');
      | if isempty(last)
      |     last = datestr(now,'yyyy');
      | else
      |     last = last(end-3:end);
      | end
      | 
      | if strcmp(first,last)
      |     fprintf('%s -- Copyright %s Nexteer',NxtrConf,first)
      | else
      |     fprintf('%s -- %s%s- %s Nexteer',NxtrConf,char(169),first,last)
      | end
  OutpAssiStHlth : Outport
  " PrsntVltgRng" : Outport  Port=2
  wires:
  Constant1/1 -> OutpAssiStHlth/1
  Constant3/1 -> " PrsntVltgRng"/1

== system ES105A_StHlthSigNormn/StHlthSigNormn/UpdRawSig/ Health Of Assist Due To Voltage/UnderVoltage ==
  Action Port : ActionPort  ActionType=elseif
  Bitwise Operator : simulink/Logic and Bit Operations/Bitwise Operator  logicop=OR  UseBitMask=off  NumInputPorts=2  BitMask=bin2dec('11011001')  BitMaskRealWorld=Stored Integer
  Constant1 : Constant  Value=HLTH0PERC_CNT_U08  OutDataTypeStr=uint8
      settings: AttributesFormatString=%<OutDataTypeStr>
  Constant2 : Constant  OutDataTypeStr=uint8
      settings: AttributesFormatString=%<OutDataTypeStr>
  Constant3 : Constant  OutDataTypeStr=uint8
      settings: AttributesFormatString=%<OutDataTypeStr>
  CopyRight2 : Subsystem  Description=|  mask(Copyright Information){none=on}
      | Copyright info block.                                               
      |                                                                     
      | Place copyright information at the top of every subsystem in design.
      mask prompts: none "No parameters"
      mask help: Place copyright information at the top of every subsystem in design.
      mask Display:
      | NxtrConf = 'Nexteer Confidential';
      | 
      | sys = bdroot; %handle for the current model ("system")
      | first = get_param(sys,'Created');
      | first = first(end-3:end);  %year is last four digits
      | 
      | last = get_param(sys,'LastModifiedDate');
      | if isempty(last)
      |     last = datestr(now,'yyyy');
      | else
      |     last = last(end-3:end);
      | end
      | 
      | if strcmp(first,last)
      |     fprintf('%s -- Copyright %s Nexteer',NxtrConf,first)
      | else
      |     fprintf('%s -- %s%s- %s Nexteer',NxtrConf,char(169),first,last)
      | end
  Data Store Read : DataStoreRead  DataStoreName=VltgRngIgnCyc
  Data Store Write : DataStoreWrite  DataStoreName=VltgRngIgnCyc
  Shift Arithmetic : ArithShift  BitShiftNumber=LOVLTGSTHLTH0PERC_CNT_U08  BitShiftDirection=Left
  Shift Arithmetic1 : ArithShift  BitShiftNumber=LOVLTGSTHLTH0PERC_CNT_U08  BitShiftDirection=Left
  OutpAssiStHlth : Outport
  " PrsntVltgRng" : Outport  Port=2
  wires:
  Constant1/1 -> OutpAssiStHlth/1
  Constant2/1 -> Shift Arithmetic/1
  Shift Arithmetic/1 -> Bitwise Operator/2
  Data Store Read/1 -> Bitwise Operator/1
  Bitwise Operator/1 -> Data Store Write/1
  Constant3/1 -> Shift Arithmetic1/1
  Shift Arithmetic1/1 -> " PrsntVltgRng"/1

== system ES105A_StHlthSigNormn/StHlthSigNormn/UpdRawSig/ Health Of Assist Due To Voltage/Voltage range update for ignition cycle ==
  Action Port : ActionPort  ActionType=then
  Bitwise Operator2 : simulink/Logic and Bit Operations/Bitwise Operator  logicop=AND  UseBitMask=off  NumInputPorts=2  BitMask=bin2dec('11011001')  BitMaskRealWorld=Stored Integer
  Constant5 : Constant  Value=VLTGSTHLTH0PERC_CNT_U08
  CopyRight2 : Subsystem  Description=|  mask(Copyright Information){none=on}
      | Copyright info block.                                               
      |                                                                     
      | Place copyright information at the top of every subsystem in design.
      mask prompts: none "No parameters"
      mask help: Place copyright information at the top of every subsystem in design.
      mask Display:
      | NxtrConf = 'Nexteer Confidential';
      | 
      | sys = bdroot; %handle for the current model ("system")
      | first = get_param(sys,'Created');
      | first = first(end-3:end);  %year is last four digits
      | 
      | last = get_param(sys,'LastModifiedDate');
      | if isempty(last)
      |     last = datestr(now,'yyyy');
      | else
      |     last = last(end-3:end);
      | end
      | 
      | if strcmp(first,last)
      |     fprintf('%s -- Copyright %s Nexteer',NxtrConf,first)
      | else
      |     fprintf('%s -- %s%s- %s Nexteer',NxtrConf,char(169),first,last)
      | end
  Data Store Read : DataStoreRead  DataStoreName=VltgRngIgnCyc
  VltgRngOut : Outport
  wires:
  Data Store Read/1 -> Bitwise Operator2/1
  Constant5/1 -> Bitwise Operator2/2
  Bitwise Operator2/1 -> VltgRngOut/1

== system ES105A_StHlthSigNormn/StHlthSigNormn/UpdRawSig/ Health Of Assist Due To Voltage/Voltage range update for ignition cycle1 ==
  Action Port : ActionPort  ActionType=else
  CopyRight2 : Subsystem  Description=|  mask(Copyright Information){none=on}
      | Copyright info block.                                               
      |                                                                     
      | Place copyright information at the top of every subsystem in design.
      mask prompts: none "No parameters"
      mask help: Place copyright information at the top of every subsystem in design.
      mask Display:
      | NxtrConf = 'Nexteer Confidential';
      | 
      | sys = bdroot; %handle for the current model ("system")
      | first = get_param(sys,'Created');
      | first = first(end-3:end);  %year is last four digits
      | 
      | last = get_param(sys,'LastModifiedDate');
      | if isempty(last)
      |     last = datestr(now,'yyyy');
      | else
      |     last = last(end-3:end);
      | end
      | 
      | if strcmp(first,last)
      |     fprintf('%s -- Copyright %s Nexteer',NxtrConf,first)
      | else
      |     fprintf('%s -- %s%s- %s Nexteer',NxtrConf,char(169),first,last)
      | end
  Data Store Read : DataStoreRead  DataStoreName=VltgRngIgnCyc
  Shift Arithmetic1 : ArithShift  BitShiftNumber=VLTGPRSNTCYCDATAPOSN_CNT_U08  BitShiftDirection=Right
  VltgRngOut : Outport
  wires:
  Data Store Read/1 -> Shift Arithmetic1/1
  Shift Arithmetic1/1 -> VltgRngOut/1

== system ES105A_StHlthSigNormn/StHlthSigNormn/UpdRawSig/ Health Of Assist Due To Voltage/Voltage range update for present cycle  ==
  PrsntVltgRng : Inport
  VltgRngOut : Inport  Port=2
  Action Port : ActionPort  ActionType=then
  Bitwise Operator : simulink/Logic and Bit Operations/Bitwise Operator  logicop=OR  UseBitMask=off  NumInputPorts=2  BitMask=bin2dec('11011001')  BitMaskRealWorld=Stored Integer
  Bitwise Operator1 : simulink/Logic and Bit Operations/Bitwise Operator  logicop=AND  UseBitMask=off  NumInputPorts=2  BitMask=bin2dec('11011001')  BitMaskRealWorld=Stored Integer
  Constant7 : Constant  Value=VLTGSTHLTH0PERC_CNT_U08
  CopyRight2 : Subsystem  Description=|  mask(Copyright Information){none=on}
      | Copyright info block.                                               
      |                                                                     
      | Place copyright information at the top of every subsystem in design.
      mask prompts: none "No parameters"
      mask help: Place copyright information at the top of every subsystem in design.
      mask Display:
      | NxtrConf = 'Nexteer Confidential';
      | 
      | sys = bdroot; %handle for the current model ("system")
      | first = get_param(sys,'Created');
      | first = first(end-3:end);  %year is last four digits
      | 
      | last = get_param(sys,'LastModifiedDate');
      | if isempty(last)
      |     last = datestr(now,'yyyy');
      | else
      |     last = last(end-3:end);
      | end
      | 
      | if strcmp(first,last)
      |     fprintf('%s -- Copyright %s Nexteer',NxtrConf,first)
      | else
      |     fprintf('%s -- %s%s- %s Nexteer',NxtrConf,char(169),first,last)
      | end
  Shift Arithmetic : ArithShift  BitShiftNumber=VLTGPRSNTCYCDATAPOSN_CNT_U08  BitShiftDirection=Left
  " VltgRng" : Outport
  wires:
  Shift Arithmetic/1 -> Bitwise Operator/2
  PrsntVltgRng/1 -> Bitwise Operator1/1
  Constant7/1 -> Bitwise Operator1/2
  Bitwise Operator1/1 -> Shift Arithmetic/1
  VltgRngOut/1 -> Bitwise Operator/1
  Bitwise Operator/1 -> " VltgRng"/1

== system ES105A_StHlthSigNormn/StHlthSigNormn/UpdRawSig/ Health Of Assist Due To Voltage/Voltage range update for present cycle1 ==
  PrsntVltgRng : Inport
  VltgRngOut : Inport  Port=2
  Action Port : ActionPort  ActionType=else
  Bitwise Operator1 : simulink/Logic and Bit Operations/Bitwise Operator  logicop=OR  UseBitMask=off  NumInputPorts=2  BitMask=bin2dec('11011001')  BitMaskRealWorld=Stored Integer
  CopyRight2 : Subsystem  Description=|  mask(Copyright Information){none=on}
      | Copyright info block.                                               
      |                                                                     
      | Place copyright information at the top of every subsystem in design.
      mask prompts: none "No parameters"
      mask help: Place copyright information at the top of every subsystem in design.
      mask Display:
      | NxtrConf = 'Nexteer Confidential';
      | 
      | sys = bdroot; %handle for the current model ("system")
      | first = get_param(sys,'Created');
      | first = first(end-3:end);  %year is last four digits
      | 
      | last = get_param(sys,'LastModifiedDate');
      | if isempty(last)
      |     last = datestr(now,'yyyy');
      | else
      |     last = last(end-3:end);
      | end
      | 
      | if strcmp(first,last)
      |     fprintf('%s -- Copyright %s Nexteer',NxtrConf,first)
      | else
      |     fprintf('%s -- %s%s- %s Nexteer',NxtrConf,char(169),first,last)
      | end
  " VltgRng" : Outport
  wires:
  PrsntVltgRng/1 -> Bitwise Operator1/1
  VltgRngOut/1 -> Bitwise Operator1/2
  Bitwise Operator1/1 -> " VltgRng"/1

== system ES105A_StHlthSigNormn/StHlthSigNormn/UpdRawSig/Controller temperature/Controller temperature range update for ignition cycle ==
  Action Port : ActionPort  ActionType=then
  Bitwise Operator2 : simulink/Logic and Bit Operations/Bitwise Operator  logicop=AND  UseBitMask=off  NumInputPorts=2  BitMask=bin2dec('11011001')  BitMaskRealWorld=Stored Integer
  Constant5 : Constant  Value=TSTHLTH0PERC_CNT_U08
  CopyRight2 : Subsystem  Description=|  mask(Copyright Information){none=on}
      | Copyright info block.                                               
      |                                                                     
      | Place copyright information at the top of every subsystem in design.
      mask prompts: none "No parameters"
      mask help: Place copyright information at the top of every subsystem in design.
      mask Display:
      | NxtrConf = 'Nexteer Confidential';
      | 
      | sys = bdroot; %handle for the current model ("system")
      | first = get_param(sys,'Created');
      | first = first(end-3:end);  %year is last four digits
      | 
      | last = get_param(sys,'LastModifiedDate');
      | if isempty(last)
      |     last = datestr(now,'yyyy');
      | else
      |     last = last(end-3:end);
      | end
      | 
      | if strcmp(first,last)
      |     fprintf('%s -- Copyright %s Nexteer',NxtrConf,first)
      | else
      |     fprintf('%s -- %s%s- %s Nexteer',NxtrConf,char(169),first,last)
      | end
  Data Store Read : DataStoreRead  DataStoreName=EcuTRngIgnCyc
  CtrlrTRngOut : Outport
  wires:
  Data Store Read/1 -> Bitwise Operator2/1
  Constant5/1 -> Bitwise Operator2/2
  Bitwise Operator2/1 -> CtrlrTRngOut/1

== system ES105A_StHlthSigNormn/StHlthSigNormn/UpdRawSig/Controller temperature/Controller temperature range update for ignition cycle1 ==
  Action Port : ActionPort  ActionType=else
  CopyRight2 : Subsystem  Description=|  mask(Copyright Information){none=on}
      | Copyright info block.                                               
      |                                                                     
      | Place copyright information at the top of every subsystem in design.
      mask prompts: none "No parameters"
      mask help: Place copyright information at the top of every subsystem in design.
      mask Display:
      | NxtrConf = 'Nexteer Confidential';
      | 
      | sys = bdroot; %handle for the current model ("system")
      | first = get_param(sys,'Created');
      | first = first(end-3:end);  %year is last four digits
      | 
      | last = get_param(sys,'LastModifiedDate');
      | if isempty(last)
      |     last = datestr(now,'yyyy');
      | else
      |     last = last(end-3:end);
      | end
      | 
      | if strcmp(first,last)
      |     fprintf('%s -- Copyright %s Nexteer',NxtrConf,first)
      | else
      |     fprintf('%s -- %s%s- %s Nexteer',NxtrConf,char(169),first,last)
      | end
  Data Store Read : DataStoreRead  DataStoreName=EcuTRngIgnCyc
  Shift Arithmetic1 : ArithShift  BitShiftNumber=TPRSNTCYCDATAPOSN_CNT_U08  BitShiftDirection=Right
  CtrlrTRngOut : Outport
  wires:
  Data Store Read/1 -> Shift Arithmetic1/1
  Shift Arithmetic1/1 -> CtrlrTRngOut/1

== system ES105A_StHlthSigNormn/StHlthSigNormn/UpdRawSig/Controller temperature/Controller temperature range update for present cycle  ==
  PrsntCtrlrTRng : Inport
  CtrlrTRngOut : Inport  Port=2
  Action Port : ActionPort  ActionType=then
  Bitwise Operator : simulink/Logic and Bit Operations/Bitwise Operator  logicop=OR  UseBitMask=off  NumInputPorts=2  BitMask=bin2dec('11011001')  BitMaskRealWorld=Stored Integer
  Bitwise Operator1 : simulink/Logic and Bit Operations/Bitwise Operator  logicop=AND  UseBitMask=off  NumInputPorts=2  BitMask=bin2dec('11011001')  BitMaskRealWorld=Stored Integer
  Constant7 : Constant  Value=TSTHLTH0PERC_CNT_U08
  CopyRight2 : Subsystem  Description=|  mask(Copyright Information){none=on}
      | Copyright info block.                                               
      |                                                                     
      | Place copyright information at the top of every subsystem in design.
      mask prompts: none "No parameters"
      mask help: Place copyright information at the top of every subsystem in design.
      mask Display:
      | NxtrConf = 'Nexteer Confidential';
      | 
      | sys = bdroot; %handle for the current model ("system")
      | first = get_param(sys,'Created');
      | first = first(end-3:end);  %year is last four digits
      | 
      | last = get_param(sys,'LastModifiedDate');
      | if isempty(last)
      |     last = datestr(now,'yyyy');
      | else
      |     last = last(end-3:end);
      | end
      | 
      | if strcmp(first,last)
      |     fprintf('%s -- Copyright %s Nexteer',NxtrConf,first)
      | else
      |     fprintf('%s -- %s%s- %s Nexteer',NxtrConf,char(169),first,last)
      | end
  Shift Arithmetic : ArithShift  BitShiftNumber=TPRSNTCYCDATAPOSN_CNT_U08  BitShiftDirection=Left
  CtrlrTRng : Outport
  wires:
  PrsntCtrlrTRng/1 -> Bitwise Operator1/1
  Constant7/1 -> Bitwise Operator1/2
  Bitwise Operator1/1 -> Shift Arithmetic/1
  Bitwise Operator/1 -> CtrlrTRng/1
  Shift Arithmetic/1 -> Bitwise Operator/1
  CtrlrTRngOut/1 -> Bitwise Operator/2

== system ES105A_StHlthSigNormn/StHlthSigNormn/UpdRawSig/Controller temperature/Controller temperature range update for present cycle1 ==
  PrsntCtrlrTRng : Inport
  CtrlrTRngOut : Inport  Port=2
  Action Port : ActionPort  ActionType=else
  Bitwise Operator1 : simulink/Logic and Bit Operations/Bitwise Operator  logicop=OR  UseBitMask=off  NumInputPorts=2  BitMask=bin2dec('11011001')  BitMaskRealWorld=Stored Integer
  CopyRight2 : Subsystem  Description=|  mask(Copyright Information){none=on}
      | Copyright info block.                                               
      |                                                                     
      | Place copyright information at the top of every subsystem in design.
      mask prompts: none "No parameters"
      mask help: Place copyright information at the top of every subsystem in design.
      mask Display:
      | NxtrConf = 'Nexteer Confidential';
      | 
      | sys = bdroot; %handle for the current model ("system")
      | first = get_param(sys,'Created');
      | first = first(end-3:end);  %year is last four digits
      | 
      | last = get_param(sys,'LastModifiedDate');
      | if isempty(last)
      |     last = datestr(now,'yyyy');
      | else
      |     last = last(end-3:end);
      | end
      | 
      | if strcmp(first,last)
      |     fprintf('%s -- Copyright %s Nexteer',NxtrConf,first)
      | else
      |     fprintf('%s -- %s%s- %s Nexteer',NxtrConf,char(169),first,last)
      | end
  CtrlrTRng : Outport
  wires:
  PrsntCtrlrTRng/1 -> Bitwise Operator1/1
  CtrlrTRngOut/1 -> Bitwise Operator1/2
  Bitwise Operator1/1 -> CtrlrTRng/1

== system ES105A_StHlthSigNormn/StHlthSigNormn/UpdRawSig/Controller temperature/CopyRight2 ==
